simulink model "Canonique_PendulumInverseSIMU_theta"  (Simulink 10.0)
settings: Solver=ode45  StartTime=ti  StopTime=tf  FixedStep=0.001  RelTol=1e-3  EnableMultiTasking=on
undefined symbols (not defined in the file): g, J, l, m, Mcart, Noise, theta
libraries: simulink x1
settings Model: Creator=huojiaxi  LastModifiedBy=huojiaxi  ExtModeTrigMode=oneshot  ExtModeArmWhenConnect=off
settings DataIOCC: SignalLoggingSaveFormat=ModelDataLogs
settings OptimizationCC: BooleanDataType=off  LifeSpan=auto
settings DebuggingCC: SaveWithParameterizedLinksMsg=none  SignalResolutionControl=TryResolveAllWithWarning  MultiTaskDSMMsg=warning  MultiTaskCondExecSysMsg=none  SFUnexpectedBacktrackingDiag=error  SFNoUnconditionalDefaultTransitionDiag=error  SFExecutionAtInitializationDiag=warning  ArithmeticOperatorsInVariantConditions=error
settings HardwareCC: ProdBitPerPointer=64  ProdBitPerSizeT=64  ProdBitPerPtrDiffT=64  ProdLargestAtomicFloat=Float  ProdIntDivRoundTo=Zero  ProdEndianess=LittleEndian  ProdWordSize=64  ProdHWDeviceType=Intel->x86-64 (Windows64)  TargetUnknown=on
settings SFSimCC: SimUseLocalCustomCode=on  CustomCodeUndefinedFunction=FilterOut
settings RTWCC: RTWUseLocalCustomCode=on
settings CodeAppCC: StateflowObjectComments=off
settings GRTTargetCC: TargetLangStandard=C99 (ISO)
settings ConfigComp: CovSaveCumulativeToWorkspaceVar=off  CovSaveSingleToWorkspaceVar=off

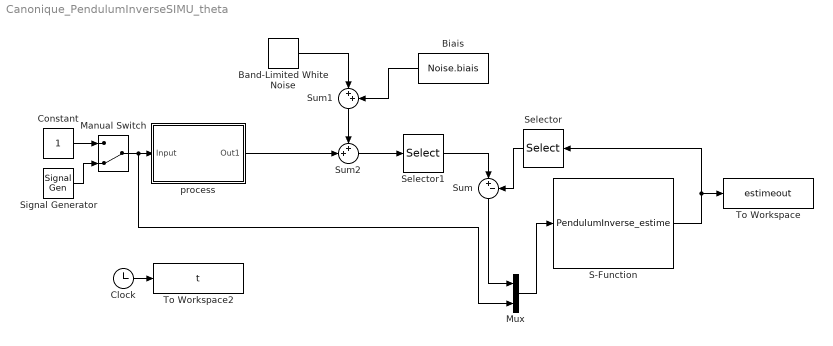
== system Canonique_PendulumInverseSIMU_theta ==
  Band-Limited White Noise : simulink/Sources/Band-Limited White Noise  Cov=Noise.power  Ts=Noise.sampling  seed=Noise.seed
  Biais : Constant  Value=Noise.biais
  Clock : Clock
  Constant : Constant
  Manual Switch : ManualSwitch  CurrentSetting=0
  Mux : Mux  Inputs=2
  S-Function : S-Function  FunctionName=PendulumInverse_estime  Parameters=Mcart,m,l,g,J,theta  SFunctionDeploymentMode=off  EnableBusSupport=off
  Selector : Selector  InputPortWidth=4  IndexOptions=Index vector (dialog)  Indices=[3]  OutputSizes=1
  Selector1 : Selector  InputPortWidth=4  IndexOptions=Index vector (dialog)  Indices=[3]  OutputSizes=1
  Signal Generator : SignalGenerator  Units=rad/sec
  Sum : Sum  Inputs=|+-
  Sum1 : Sum  Inputs=|++
  Sum2 : Sum  Inputs=++|
  To Workspace : ToWorkspace  VariableName=estimeout  SampleTime=-1
  To Workspace2 : ToWorkspace  VariableName=t  SampleTime=-1
  process : Subsystem
  wires:
  Sum1/1 -> Sum2/1
  Biais/1 -> Sum1/2
  Band-Limited White Noise/1 -> Sum1/1
  Sum2/1 -> Selector1/1
  process/1(Out1) -> Sum2/2
  Clock/1 -> To Workspace2/1
  Manual Switch/1 -> Mux/2, process/1(Input)
  Constant/1 -> Manual Switch/1
  Signal Generator/1 -> Manual Switch/2
  S-Function/1 -> Selector/1, To Workspace/1
  Selector1/1 -> Sum/1
  Selector/1 -> Sum/2
  Sum/1 -> Mux/1
  Mux/1 -> S-Function/1

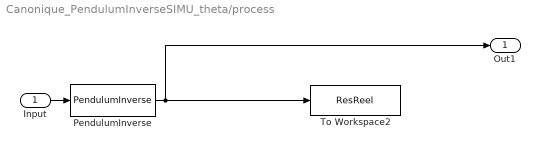
== system Canonique_PendulumInverseSIMU_theta/process ==
  Input : Inport
  PendulumInverse : S-Function  FunctionName=PendulumInverse  Parameters=Mcart,m,l,g,J  SFunctionDeploymentMode=off  EnableBusSupport=off
  To Workspace2 : ToWorkspace  VariableName=ResReel  SampleTime=-1
  Out1 : Outport
  wires:
  Input/1 -> PendulumInverse/1
  PendulumInverse/1 -> To Workspace2/1, Out1/1
